simulink model "autosar_tpc_throttle_sensor_monitor"  (R2022a)
settings: Solver=FixedStepDiscrete  StartTime=0.0  StopTime=10.0  FixedStep=0.005  RelTol=1e-3
undefined symbols (not defined in the file or in its folder): Dem_EventStatusType
libraries: autosarlibdem x5
settings Model: Creator=The MathWorks, Inc.  LastModifiedBy=tsen
settings SolverCC: AlgebraicLoopSolver=TrustRegion
settings DataIOCC: ReturnWorkspaceOutputs=off
settings OptimizationCC: DefaultParameterBehavior=Inlined  PassReuseOutputArgsAs=Individual arguments  ZeroExternalMemoryAtStartup=off  ZeroInternalMemoryAtStartup=off  EfficientTunableParamExpr=on
settings DebuggingCC: ParameterTunabilityLossMsg=error  UnconnectedInputMsg=warning  UnconnectedOutputMsg=warning  UnconnectedLineMsg=warning  SFMachineParentedDataDiag=warning  ArithmeticOperatorsInVariantConditions=warning
settings SFSimCC: SimUseLocalCustomCode=off  MATLABDynamicMemAlloc=off
settings RTWCC: Description=AUTOSAR  SystemTargetFile=autosar.tlc  GenCodeOnly=on  TemplateMakefile=ert_default_tmf  GenerateReport=on  RTWVerbose=off  RTWUseLocalCustomCode=off  IncludeHyperlinkInReport=on  LaunchReport=on  GenerateTraceInfo=on  GenerateTraceReport=on  GenerateTraceReportSl=on  GenerateTraceReportSf=on  GenerateTraceReportEml=on
settings CodeAppCC: ForceParamTrailComments=on  IgnoreCustomStorageClasses=off  OperatorAnnotations=on  SimulinkDataObjDesc=on  SFDataObjDesc=on  InsertBlockDesc=on
settings STFCustomTargetCC: TargetLangStandard=C99 (ISO)  MultiwordLength=256  ParMdlRefBuildCompliant=on  CompOptLevelCompliant=on  IncludeMdlTerminateFcn=off  CombineOutputUpdateFcns=on  SuppressErrorStatus=on  ERTCustomFileBanners=on  SupportNonFinite=off  SupportComplex=off  SupportContinuousTime=off  SupportNonInlinedSFcns=off  RemoveResetFunc=on  MATLABClassNameForMDSCustomization=Simulink.SoftwareTarget.ERTCustomization  AutosarCompliant=on  GRTInterface=off  UseToolchainInfoCompliant=on  LookupTableObjectStructAxisOrder=2,1,3,4,...  LUTObjectStructOrderEvenSpacing=Size,Table,Breakpoints  SystemTargetFile=autosar.tlc
settings ERTTargetCC: TargetLangStandard=C99 (ISO)  ConcurrentExecutionCompliant=off  IncludeMdlTerminateFcn=off  SuppressErrorStatus=on  SupportNonFinite=off  SupportComplex=off  ModelStepFunctionPrototypeControlCompliant=off  CPPClassGenCompliant=off  AutosarCompliant=on  LookupTableObjectStructAxisOrder=2,1,3,4,...  LUTObjectStructOrderEvenSpacing=Size,Table,Breakpoints  InlinedParameterPlacement=NonHierarchical  ERTCustomFileTemplate=example_file_process.tlc

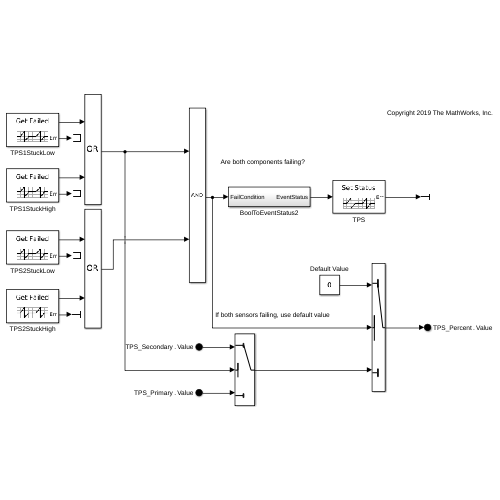
[thumbnail: Simulink's stored preview of the top-level diagram]
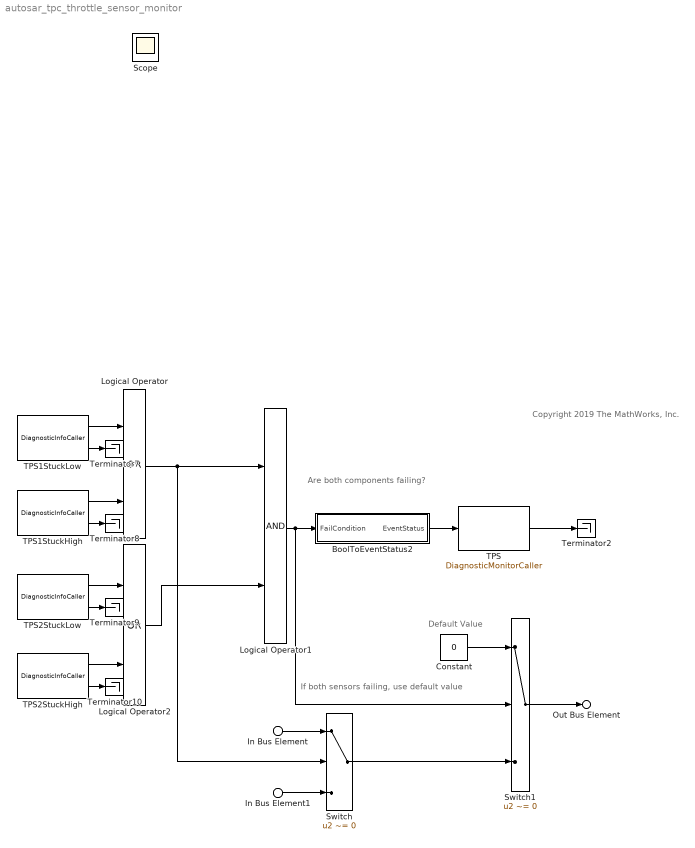
== system autosar_tpc_throttle_sensor_monitor ==
  note: Default Value
  note: Are both components failing?
  note: If both sensors failing, use default value
  note: Copyright 2019 The MathWorks, Inc.
  In Bus Element1 : Inport  PortName=TPS_Primary  Element=Value
  In Bus Element : Inport  Port=2  PortName=TPS_Secondary  Element=Value
  BoolToEventStatus2 : Subsystem
  Constant : Constant  Value=0  OutDataTypeStr=single
  Logical Operator : Logic  Operator=OR  AllPortsSameDT=off  OutDataTypeStr=boolean
  Logical Operator1 : Logic  AllPortsSameDT=off  OutDataTypeStr=boolean
  Logical Operator2 : Logic  Operator=OR  AllPortsSameDT=off  OutDataTypeStr=boolean
  Switch : Switch  Criteria=u2 ~= 0  SaturateOnIntegerOverflow=off  InputSameDT=off
  Switch1 : Switch  Criteria=u2 ~= 0  SaturateOnIntegerOverflow=off  InputSameDT=off
  TPS : autosarlibdem/DiagnosticMonitorCaller  PortName=TPS  Operation=SetEventStatus  Datatype=Enum: Dem_EventStatusType  st=-1  ServiceImpl=autosar.bsw.DemDiagnosticMonitor
      settings: SourceProductBaseCode=AS
  TPS1StuckHigh : autosarlibdem/DiagnosticInfoCaller  PortName=TPS1StuckHigh  Operation=GetEventFailed  st=.005  ServiceImpl=autosar.bsw.DemDiagnosticInfo
      settings: SourceProductBaseCode=AS
  TPS1StuckLow : autosarlibdem/DiagnosticInfoCaller  PortName=TPS1StuckLow  Operation=GetEventFailed  st=.005  ServiceImpl=autosar.bsw.DemDiagnosticInfo
      settings: SourceProductBaseCode=AS
  TPS2StuckHigh : autosarlibdem/DiagnosticInfoCaller  PortName=TPS2StuckHigh  Operation=GetEventFailed  st=.005  ServiceImpl=autosar.bsw.DemDiagnosticInfo
      settings: SourceProductBaseCode=AS
  TPS2StuckLow : autosarlibdem/DiagnosticInfoCaller  PortName=TPS2StuckLow  Operation=GetEventFailed  st=.005  ServiceImpl=autosar.bsw.DemDiagnosticInfo
      settings: SourceProductBaseCode=AS
  Terminator{2,7..10} (5 alike) : Terminator
  Out Bus Element : Outport  VectorParamsAs1DForOutWhenUnconnected=off  PortName=TPS_Percent  Element=Value
  Scope : Scope
  wires:
  TPS1StuckLow/1 -> Logical Operator/1
  TPS/1 -> Terminator2/1
  BoolToEventStatus2/1(EventStatus) -> TPS/1
  Logical Operator/1 -> Switch/2, Logical Operator1/1
  TPS1StuckHigh/1 -> Logical Operator/2
  Constant/1 -> Switch1/1
  Switch/1 -> Switch1/3
  TPS2StuckLow/2 -> Terminator9/1
  Logical Operator2/1 -> Logical Operator1/2
  TPS1StuckHigh/2 -> Terminator8/1
  TPS2StuckHigh/1 -> Logical Operator2/2
  TPS2StuckHigh/2 -> Terminator10/1
  Logical Operator1/1 -> Switch1/2, BoolToEventStatus2/1(FailCondition)
  TPS1StuckLow/2 -> Terminator7/1
  TPS2StuckLow/1 -> Logical Operator2/1
  In Bus Element/1 -> Switch/1
  In Bus Element1/1 -> Switch/3
  Switch1/1 -> Out Bus Element/1

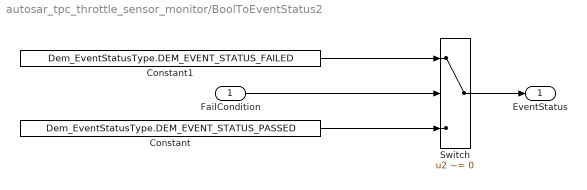
== system autosar_tpc_throttle_sensor_monitor/BoolToEventStatus2 ==
  FailCondition : Inport
  Constant : Constant  Value=Dem_EventStatusType.DEM_EVENT_STATUS_PASSED
  Constant1 : Constant  Value=Dem_EventStatusType.DEM_EVENT_STATUS_FAILED
  Switch : Switch  Criteria=u2 ~= 0  SaturateOnIntegerOverflow=off  InputSameDT=off
  EventStatus : Outport  VectorParamsAs1DForOutWhenUnconnected=off
  wires:
  Switch/1 -> EventStatus/1
  Constant1/1 -> Switch/1
  Constant/1 -> Switch/3
  FailCondition/1 -> Switch/2
